simulink model "psbsimplealt"  (Simulink 6.0)
settings: Solver=ode23tb  SolverMode=SingleTasking  StartTime=0.0  StopTime=2  FixedStep=1e-3  RelTol=1e-3
libraries: powerlib2 x9, powerlib_extras x2
settings Model: Creator=patrice  LastModifiedBy=batserve  ExtModeTrigMode=oneshot  ExtModeArmWhenConnect=off  ExtModeAutoUpdateStatusClock=off
settings DataIOCC: InitialState=xinit  LimitDataPoints=off  SaveOutput=off  TimeSaveName=t  SignalLoggingName=sigsOut
settings OptimizationCC: BooleanDataType=off
settings DebuggingCC: SolverPrmCheckMsg=none  UnconnectedInputMsg=none  UnconnectedOutputMsg=none
settings HardwareCC: TargetUnknown=on
settings RTWCC: TemplateMakefile=grt_unix.tmf

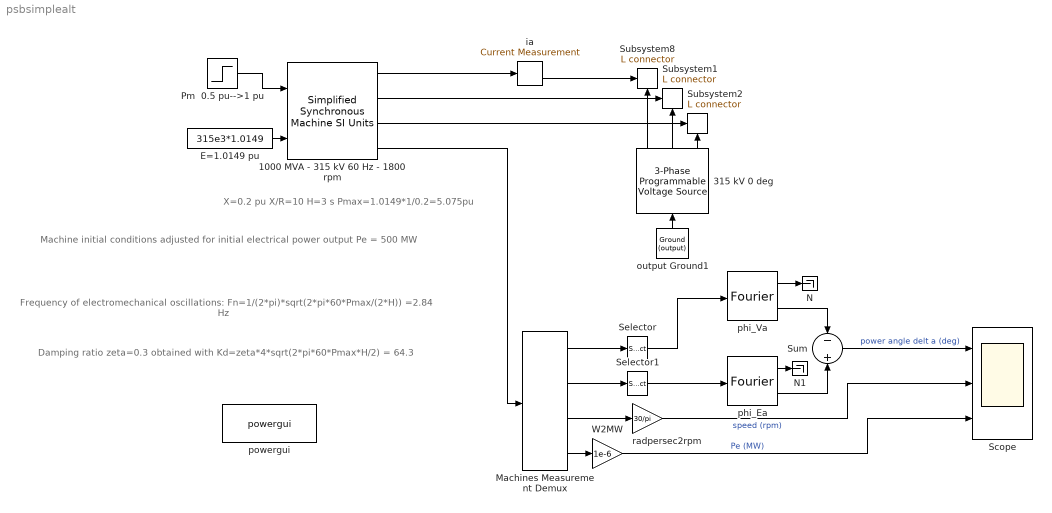
== system psbsimplealt ==
  note: Machine  initial conditions adjusted
      | for initial  electrical power output Pe = 500 MW
  note: X=0.2 pu X/R=10 H=3 s Pmax=1.0149*1/0.2=5.075pu
  note: Frequency of electromechanical oscillations:
      | Fn=1/(2*pi)*sqrt(2*pi*60*Pmax/(2*H)) =2.84 Hz
  note: Damping ratio zeta=0.3 obtained with
      | Kd=zeta*4*sqrt(2*pi*60*Pmax*H/2) = 64.3
  1000 MVA - 315 kV 60 Hz - 1800 rpm : powerlib2/Machines/Simplified Synchronous  Machine SI Units  Tag=PoWeRsYsTeMbLoCk  conType=3-wire Y  x1=[ 1000e6, 315e3, 60 ]  x2="[168870,  64.3,  2]"  x3=[ 99.225*0.02 ,99.225/(2*pi*60)*0.2 ]  x4=[0 5.65442 1296.03 1296.03 1296.03 0 -120 120]  PSBOutputType=1110  iounits=1  LoadFlowParameters=[1 500000000 0 0 0]
  315 kV 0 deg : powerlib2/Electrical Sources/3-Phase  Programmable  Voltage Source  Orientation=up  Par_Vps_LLrms="[315e3 0  60]"  VariationEntity=None  VariationType=Step  VariationStep=-0.5  VariationRate=10  VariationMag=0.3  VariationFreq=2  Par_Timing_Variation=[0.1 1.2]  SinglePhase=off  Yampli=[1 0.8 1.2 1.0]  Xtime=[0 0.1 0.15 0.2]  HarmonicGeneration=off  Par_HarmoA_pu=[3 0.2 -25 0]  Par_HarmoB_pu="[2 0.15  35 2]"  Par_Timing_Harmo="[0.05  3]"
  E=1.0149 pu : Constant  Value=315e3*1.0149
  Machines Measurement Demux : powerlib2/Machines/Machines Measurement Demux  machType=Simplified synchronous  ssm1=off  ssm2=on  ssm3=on  ssm4=off  ssm5=on  ssm6=on  sm1=on  sm2=on  sm3=on  sm4=on  sm5=on  sm6=on  sm7=on  sm8=on  sm9=on  sm10=on  sm11=off  sm115=off  sm12=off  sm13=off  sm14=off  asm1=on  asm2=on  asm3=on  asm4=on  asm5=on  asm6=on  asm7=on  asm8=on  asm9=on  asm10=on  asm11=on  pmsm1=on  pmsm2=on  pmsm3=on  pmsm4=on  pmsm5=on  pmsm6=on  lastType=1
  N : Terminator
  N1 : Terminator
  Pm  0.5 pu-->1 pu : Step  Time=0.5  Before=505e6  After=1000e6  SampleTime=0
  Scope : Scope  NumInputPorts=3
      settings: YMin=5~1797~500  YMax=14~1806~1200  SaveName=delta  DataFormat=Structure
  Selector : Selector  InputPortWidth=3
  Selector1 : Selector  InputPortWidth=3
  Subsystem1 : powerlib2/Connectors/L connector  Tag=PoWeRsYsTeMbLoCk  Orientation=up
  Subsystem2 : powerlib2/Connectors/L connector  Tag=PoWeRsYsTeMbLoCk  Orientation=up
  Subsystem8 : powerlib2/Connectors/L connector  Tag=PoWeRsYsTeMbLoCk  Orientation=up
  Sum : Sum  Inputs=-+  SaturateOnIntegerOverflow=on  InputSameDT=on
  W2MW : Gain  Gain=1e-6  SaturateOnIntegerOverflow=on
  ia : powerlib2/Measurements/Current Measurement  Tag=PoWeRsYsTeMmEaSuReMeNt  PhasorSimulation=off  OutputType=Magnitude  PSBOutputType=01  PSBequivalent=0
  output Ground1 : powerlib2/Connectors/Ground (output)  Tag=PoWeRsYsTeMbLoCk  Orientation=up  PSBOutputType=1
  phi_Ea : powerlib_extras/Measurements/Fourier  f1=60  n=1
  phi_Va : powerlib_extras/Measurements/Fourier  f1=60  n=1
  powergui : powerlib2/powergui  Frange=[0:2:500]  Ylog=off  Xlog=off  save=off  variable=ZData  ZoomFFT=on  StartTime=0.0  cycles=1  DisplayStyle=off  fundamental=60  FreqAxis=off  MaxFrequency=1000  frequencyindice=60  frequencyindicesteady=1  RmsSteady=1  display=off  Ts=0  methode=off  frequency=60  echomessages=off
  radpersec2rpm : Gain  Gain=30/pi  SaturateOnIntegerOverflow=on
  wires:
  Pm  0.5 pu-->1 pu/1 -> 1000 MVA - 315 kV 60 Hz - 1800 rpm/1
  E=1.0149 pu/1 -> 1000 MVA - 315 kV 60 Hz - 1800 rpm/2
  1000 MVA - 315 kV 60 Hz - 1800 rpm/4 -> Machines Measurement Demux/1
  1000 MVA - 315 kV 60 Hz - 1800 rpm/1 -> ia/1
  1000 MVA - 315 kV 60 Hz - 1800 rpm/3 -> Subsystem2/Enable
  Machines Measurement Demux/1 -> Selector/1
  Machines Measurement Demux/2 -> Selector1/1
  Selector1/1 -> phi_Ea/1
  Selector/1 -> phi_Va/1
  Machines Measurement Demux/3 -> radpersec2rpm/1
  radpersec2rpm/1 -> Scope/2  "speed (rpm)"
  Machines Measurement Demux/4 -> W2MW/1
  W2MW/1 -> Scope/3  "Pe (MW)"
  phi_Va/2 -> Sum/1
  phi_Ea/2 -> Sum/2
  Sum/1 -> Scope/1  "power angle delt a (deg)"
  phi_Va/1 -> N/1
  phi_Ea/1 -> N1/1
  output Ground1/1 -> 315 kV 0 deg/1
  ia/2 -> Subsystem8/Enable
  315 kV 0 deg/1 -> Subsystem8/1
  1000 MVA - 315 kV 60 Hz - 1800 rpm/2 -> Subsystem1/Enable
  315 kV 0 deg/2 -> Subsystem1/1
  315 kV 0 deg/3 -> Subsystem2/1
